simulink model "ALL_IN_ONE"  (R2024b)
settings: Solver=VariableStepAuto  StartTime=0.0  StopTime=0.6  RelTol=1e-3
undefined symbols (not defined in the file or in its folder): sigbuilder_block
libraries: spsSeriesRLCBranchLib x16, spsCurrentMeasurementLib x4, spsDiodeLib x4, spsPWMGeneratorDCDCLib x4, spsMosfetLib x4, spsPVArrayLib x4, spsVoltageMeasurementLib x4, fuzblock x1, deeplib x1, slpidlib x1, spspowerguiLib x1
settings Model: Creator=RASITH  LastModifiedBy=RASITH

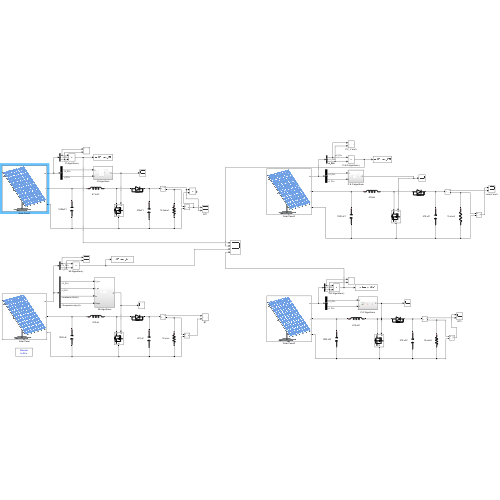
[thumbnail: Simulink's stored preview of the top-level diagram]
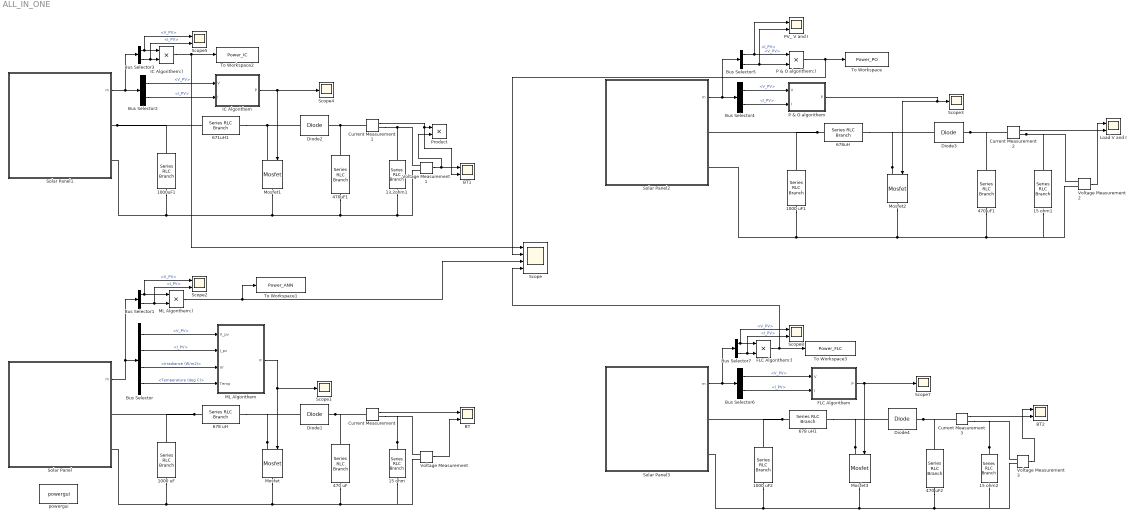
== system ALL_IN_ONE ==
  1000 uF : spsSeriesRLCBranchLib/Series RLC Branch  LConnTagsString=__new0  RConnTagsString=__new0  BranchType=C  Resistance=1  Inductance=1e-3  SetiL0=off  InitialCurrent=0  Capacitance=1e-3  Setx0=off  InitialVoltage=0  Measurements=None
  1000 uF1 : spsSeriesRLCBranchLib/Series RLC Branch  LConnTagsString=__new0  RConnTagsString=__new0  BranchType=C  Resistance=1  Inductance=1e-3  SetiL0=off  InitialCurrent=0  Capacitance=1e-3  Setx0=off  InitialVoltage=0  Measurements=None
  1000 uF2 : spsSeriesRLCBranchLib/Series RLC Branch  LConnTagsString=__new0  RConnTagsString=__new0  BranchType=C  Resistance=1  Inductance=1e-3  SetiL0=off  InitialCurrent=0  Capacitance=1e-3  Setx0=off  InitialVoltage=0  Measurements=None
  1000uF1 : spsSeriesRLCBranchLib/Series RLC Branch  LConnTagsString=__new0  RConnTagsString=__new0  BranchType=C  Resistance=1  Inductance=1e-3  SetiL0=off  InitialCurrent=0  Capacitance=1e-3  Setx0=off  InitialVoltage=0  Measurements=None
  13.2ohm1 : spsSeriesRLCBranchLib/Series RLC Branch  LConnTagsString=__new0  RConnTagsString=__new0  BranchType=R  Resistance=30  Inductance=1e-3  SetiL0=off  InitialCurrent=0  Capacitance=1e-6  Setx0=off  InitialVoltage=0  Measurements=None
  15 ohm : spsSeriesRLCBranchLib/Series RLC Branch  LConnTagsString=__new0  RConnTagsString=__new0  BranchType=R  Resistance=30  Inductance=1e-3  SetiL0=off  InitialCurrent=0  Capacitance=1e-6  Setx0=off  InitialVoltage=0  Measurements=Branch voltage and current
  15 ohm1 : spsSeriesRLCBranchLib/Series RLC Branch  LConnTagsString=__new0  RConnTagsString=__new0  BranchType=R  Resistance=30  Inductance=1e-3  SetiL0=off  InitialCurrent=0  Capacitance=1e-6  Setx0=off  InitialVoltage=0  Measurements=None
  15 ohm2 : spsSeriesRLCBranchLib/Series RLC Branch  LConnTagsString=__new0  RConnTagsString=__new0  BranchType=R  Resistance=17  Inductance=1e-3  SetiL0=off  InitialCurrent=0  Capacitance=1e-6  Setx0=off  InitialVoltage=0  Measurements=None
  470 uF : spsSeriesRLCBranchLib/Series RLC Branch  LConnTagsString=__new0  RConnTagsString=__new0  BranchType=C  Resistance=1  Inductance=1e-3  SetiL0=off  InitialCurrent=0  Capacitance=470e-6  Setx0=off  InitialVoltage=0  Measurements=None
  470 uF1 : spsSeriesRLCBranchLib/Series RLC Branch  LConnTagsString=__new0  RConnTagsString=__new0  BranchType=C  Resistance=1  Inductance=1e-3  SetiL0=off  InitialCurrent=0  Capacitance=470e-6  Setx0=off  InitialVoltage=0  Measurements=None
  470 uF2 : spsSeriesRLCBranchLib/Series RLC Branch  LConnTagsString=__new0  RConnTagsString=__new0  BranchType=C  Resistance=1  Inductance=1e-3  SetiL0=off  InitialCurrent=0  Capacitance=470e-6  Setx0=off  InitialVoltage=40  Measurements=None
  470uF1 : spsSeriesRLCBranchLib/Series RLC Branch  LConnTagsString=__new0  RConnTagsString=__new0  BranchType=C  Resistance=1  Inductance=1e-3  SetiL0=off  InitialCurrent=0  Capacitance=470e-6  Setx0=off  InitialVoltage=0  Measurements=None
  671uH1 : spsSeriesRLCBranchLib/Series RLC Branch  LConnTagsString=__new0  RConnTagsString=__new0  BranchType=L  Resistance=1  Inductance=678e-6  SetiL0=off  InitialCurrent=0  Capacitance=1e-6  Setx0=off  InitialVoltage=0  Measurements=None
  678 uH : spsSeriesRLCBranchLib/Series RLC Branch  LConnTagsString=__new0  RConnTagsString=__new0  BranchType=L  Resistance=1  Inductance=678e-6  SetiL0=off  InitialCurrent=0  Capacitance=1e-6  Setx0=off  InitialVoltage=0  Measurements=None
  678 uH1 : spsSeriesRLCBranchLib/Series RLC Branch  LConnTagsString=__new0  RConnTagsString=__new0  BranchType=L  Resistance=1  Inductance=678e-6  SetiL0=off  InitialCurrent=0  Capacitance=1e-6  Setx0=off  InitialVoltage=0  Measurements=None
  678uH : spsSeriesRLCBranchLib/Series RLC Branch  LConnTagsString=__new0  RConnTagsString=__new0  BranchType=L  Resistance=1  Inductance=678e-6  SetiL0=off  InitialCurrent=0  Capacitance=1e-6  Setx0=off  InitialVoltage=0  Measurements=None
  BT : Scope  NumInputPorts=2
  BT1 : Scope  NumInputPorts=2
  BT2 : Scope  NumInputPorts=2
  Bus Selector : BusSelector  OutputSignals=V_PV,I_PV,Irradiance (W/m2),Temperature (deg C)
  Bus Selector{1..7} (7 alike) : BusSelector  OutputSignals=V_PV,I_PV
  Current Measurement{,1..3} (4 alike) : spsCurrentMeasurementLib/Current Measurement  PhasorSimulation=off  OutputType=Complex  PSBequivalent=0
  Diode{1..4} (4 alike) : spsDiodeLib/Diode  Ron=0.001  Lon=0  Vf=0.8  IC=0  UseSnubber=0  Rs=500  Cs=250e-9  Measurements=off
  FLC Algorithem : Subsystem
  FLC Algorithem:) : Product
  IC Algorithem : Subsystem
  IC Algorithem:) : Product
  Load V and I : Scope  NumInputPorts=2
  ML Algorithem : Subsystem
  ML Algorithem:) : Product
  Mosfet : spsMosfetLib/Mosfet  Ron=4.2e-3  Lon=0  Rd=0.01  Vfd=0  IC=0  Rs=1e5  Cs=1e-9  Measurements=off
  Mosfet1 : spsMosfetLib/Mosfet  Ron=4.2e-3  Lon=0  Rd=0.01  Vfd=0  IC=0  Rs=1e5  Cs=1e-9  Measurements=off
  Mosfet2 : spsMosfetLib/Mosfet  Ron=4.2e-3  Lon=0  Rd=0.01  Vfd=1  IC=0  Rs=1e5  Cs=1e-9  Measurements=off
  Mosfet3 : spsMosfetLib/Mosfet  Ron=4.2e-3  Lon=0  Rd=0.01  Vfd=0  IC=0  Rs=1e5  Cs=1e-9  Measurements=off
  P & O algorithem : Subsystem
  P & O algorithem:) : Product
  PV_ V and I : Scope  NumInputPorts=2
  Product : Product
  Scope : Scope  NumInputPorts=4
  Scope{1,3..4,7} (4 alike) : Scope
  Scope2 : Scope  NumInputPorts=2
  Scope5 : Scope  NumInputPorts=2
  Scope8 : Scope  NumInputPorts=2
  Solar Panel : Subsystem
      mask Display: image('C:\Users\RASITH\MATLAB Drive\Final Year Project [MPPT Boost Converter(PV)]\Solar Panel.png');
  Solar Panel1 : Subsystem
      mask Display: image('C:\Users\RASITH\MATLAB Drive\Final Year Project [MPPT Boost Converter(PV)]\Solar Panel.png');
  Solar Panel2 : Subsystem
      mask Display: image('C:\Users\RASITH\MATLAB Drive\Final Year Project [MPPT Boost Converter(PV)]\Solar Panel.png');
  Solar Panel3 : Subsystem
      mask Display: image('C:\Users\RASITH\MATLAB Drive\Final Year Project [MPPT Boost Converter(PV)]\Solar Panel.png');
  To Workspace : ToWorkspace  VariableName=Power_PO  SaveFormat=Timeseries  SampleTime=-1
  To Workspace1 : ToWorkspace  VariableName=Power_ANN  SaveFormat=Timeseries  SampleTime=-1
  To Workspace2 : ToWorkspace  VariableName=Power_IC  SaveFormat=Timeseries  SampleTime=-1
  To Workspace3 : ToWorkspace  VariableName=Power_FLC  SaveFormat=Timeseries  SampleTime=-1
  Voltage Measurement{,1..3} (4 alike) : spsVoltageMeasurementLib/Voltage Measurement  PhasorSimulation=off  OutputType=Complex  PSBequivalent=0
  powergui : spspowerguiLib/powergui  Priority=1  SimulationMode=Discrete  SampleTime=1e-6  frequency=100000  Iterations=50  frequencyindice=0  Pbase=100e6  ErrMax=1e-4  UnitsV=kV  UnitsW=MW  buscounter=0  FunctionMessages=off  echomessages=off  EnableUseOfTLC=off  CurrentSourceSwitches=off  DisableSnubberDevices=off  DisableRonSwitches=off  DisableVfSwitches=off  DisplayEquations=off  AutomaticDiscreteSolvers=off  SolverType=Tustin/Backward Euler (TBE)  Interpol=off  ExternalGateDelay=off  methode=off  Ts=100  x0status=blocks  SPID=on  SwTol=0  HookPort=off  NonlinearTolerance=1e-4  nMaxIteration=100  ContinueOnMaxIteration=off  RestoreLinks=warning  ResistiveCurrentMeasurement=off  Frange=[0:2:500]  Ylog=off  Xlog=on  ShowGrid=off  save=off  variable=ZData  structure=0  ZoomFFT=off  StartTime=0.0  cycles=1  DisplayStyle=1  fundamental=60  FreqAxis=off  MaxFrequency=1000  frequencyindicesteady=1  RmsSteady=1  display=off
  wires:
  Bus Selector3/1 -> Scope5/1, IC Algorithem:)/1  "<V_PV>"
  Bus Selector/3 -> ML Algorithem/3(Irr)  "<Irradiance (W/m2)>"
  Current Measurement/1 -> BT/1
  Bus Selector3/2 -> Scope5/2, IC Algorithem:)/2  "<I_PV>"
  ML Algorithem:)/1 -> To Workspace1/1, Scope/3
  Current Measurement1/1 -> BT1/2, Product/1
  Voltage Measurement1/1 -> Product/2, BT1/1
  Bus Selector/1 -> ML Algorithem/1(V_pv)  "<V_PV>"
  Bus Selector2/2 -> IC Algorithem/2(I)  "<I_PV>"
  Solar Panel1/1(m) -> Bus Selector3/1, Bus Selector2/1
  IC Algorithem/1(P) -> Scope4/1, Mosfet1/1
  Voltage Measurement/1 -> BT/2
  Bus Selector/4 -> ML Algorithem/4(Temp)  "<Temperature (deg C)>"
  Bus Selector1/2 -> Scope2/2, ML Algorithem:)/2  "<I_PV>"
  Bus Selector1/1 -> Scope2/1, ML Algorithem:)/1  "<V_PV>"
  ML Algorithem/1(P) -> Mosfet/1, Scope1/1
  Solar Panel/1(m) -> Bus Selector1/1, Bus Selector/1
  Bus Selector/2 -> ML Algorithem/2(I_pv)  "<I_PV>"
  Bus Selector2/1 -> IC Algorithem/1(V)  "<V_PV>"
  IC Algorithem:)/1 -> To Workspace2/1, Scope/1
  Bus Selector4/1 -> P & O algorithem/1(V)  "<V_PV>"
  Current Measurement2/1 -> Load V and I/2
  Bus Selector4/2 -> P & O algorithem/2(I)  "<I_PV>"
  Bus Selector5/1 -> PV_ V and I/1, P & O algorithem:)/1  "<V_PV>"
  Bus Selector5/2 -> P & O algorithem:)/2, PV_ V and I/2  "<I_PV>"
  P & O algorithem/1(P) -> Scope3/1, Mosfet2/1
  Solar Panel2/1(m) -> Bus Selector5/1, Bus Selector4/1
  Voltage Measurement2/1 -> Load V and I/1
  Solar Panel3/1(m) -> Bus Selector7/1, Bus Selector6/1
  Bus Selector6/1 -> FLC Algorithem/1(V)  "<V_PV>"
  FLC Algorithem/1(P) -> Scope7/1, Mosfet3/1
  Voltage Measurement3/1 -> BT2/1
  Current Measurement3/1 -> BT2/2
  Bus Selector7/1 -> Scope8/1, FLC Algorithem:)/1  "<V_PV>"
  Bus Selector6/2 -> FLC Algorithem/2(I)  "<I_PV>"
  Bus Selector7/2 -> Scope8/2, FLC Algorithem:)/2  "<I_PV>"
  FLC Algorithem:)/1 -> To Workspace3/1, Scope/4
  P & O algorithem:)/1 -> To Workspace/1, Scope/2
  connections:
  678 uH/LConn1 -- 1000 uF/LConn1 -- Solar Panel/RConn1
  Mosfet/RConn1 -- 15 ohm/RConn1 -- Voltage Measurement/LConn2 -- 470 uF/RConn1 -- 1000 uF/RConn1 -- Solar Panel/RConn2
  Mosfet/LConn1 -- 678 uH/RConn1 -- Diode1/LConn1
  Solar Panel1/RConn1 -- 671uH1/LConn1 -- 1000uF1/LConn1
  Current Measurement1/RConn1 -- 13.2ohm1/LConn1 -- Voltage Measurement1/LConn1
  Diode2/LConn1 -- Mosfet1/LConn1 -- 671uH1/RConn1
  Current Measurement1/LConn1 -- Diode2/RConn1 -- 470uF1/LConn1
  Voltage Measurement1/LConn2 -- 13.2ohm1/RConn1 -- 470uF1/RConn1 -- 1000uF1/RConn1 -- Solar Panel1/RConn2 -- Mosfet1/RConn1
  Diode1/RConn1 -- 470 uF/LConn1 -- Current Measurement/LConn1
  15 ohm/LConn1 -- Voltage Measurement/LConn1 -- Current Measurement/RConn1
  678uH/LConn1 -- 1000 uF1/LConn1 -- Solar Panel2/RConn1
  Mosfet2/RConn1 -- 1000 uF1/RConn1 -- Solar Panel2/RConn2 -- 15 ohm1/RConn1 -- Voltage Measurement2/LConn2 -- 470 uF1/RConn1
  Mosfet2/LConn1 -- 678uH/RConn1 -- Diode3/LConn1
  Diode3/RConn1 -- Current Measurement2/LConn1 -- 470 uF1/LConn1
  Current Measurement2/RConn1 -- Voltage Measurement2/LConn1 -- 15 ohm1/LConn1
  15 ohm2/LConn1 -- Voltage Measurement3/LConn1 -- Current Measurement3/RConn1
  Mosfet3/RConn1 -- Voltage Measurement3/LConn2 -- 15 ohm2/RConn1 -- 470 uF2/RConn1 -- 1000 uF2/RConn1 -- Solar Panel3/RConn2
  Mosfet3/LConn1 -- 678 uH1/RConn1 -- Diode4/LConn1
  Diode4/RConn1 -- 470 uF2/LConn1 -- Current Measurement3/LConn1
  678 uH1/LConn1 -- 1000 uF2/LConn1 -- Solar Panel3/RConn1

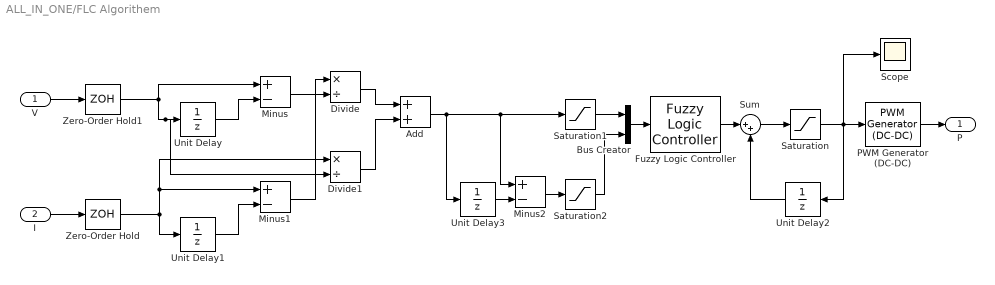
== system ALL_IN_ONE/FLC Algorithem ==
  V : Inport
  I : Inport  Port=2
  Add : Sum
  Bus Creator : BusCreator  Inputs=2
  Divide : Product  Inputs=*/
  Divide1 : Product  Inputs=*/
  Fuzzy Logic Controller : fuzblock/Fuzzy Logic  Controller  FIS=mamdani  OutputSampleNumber=49  DataType=double  FuzzifiedInputs=off  RuleFiringStrengths=off  RuleOutputs=off  AggregatedOutputs=off  SimulateUsing=Interpreted execution  OutOfRangeInputValueMessage=warning  NoRuleFiredMessage=warning  EmptyOutputFuzzySetMessage=warning
  Minus : Sum  Inputs=+-
  Minus1 : Sum  Inputs=+-
  Minus2 : Sum  Inputs=+-
  PWM Generator (DC-DC) : spsPWMGeneratorDCDCLib/PWM Generator (DC-DC)  Fsw=10000  Ts=1e-6
  Saturation : Saturate  UpperLimit=0.9  LowerLimit=0.1
  Saturation1 : Saturate  UpperLimit=1.5  LowerLimit=-1.5
  Saturation2 : Saturate  UpperLimit=0.02  LowerLimit=-0.02
  Scope : Scope
  Sum : Sum  Inputs=|++
  Unit Delay{,1..3} (4 alike) : UnitDelay  SampleTime=-1  HasFrameUpgradeWarning=on
  Zero-Order Hold : ZeroOrderHold  SampleTime=1e-3
  Zero-Order Hold1 : ZeroOrderHold  SampleTime=1e-3
  P : Outport
  wires:
  I/1 -> Zero-Order Hold/1
  V/1 -> Zero-Order Hold1/1
  Bus Creator/1 -> Fuzzy Logic Controller/1
  Fuzzy Logic Controller/1 -> Sum/1
  Sum/1 -> Saturation/1
  Saturation/1 -> Scope/1, PWM Generator (DC-DC)/1, Unit Delay2/1
  Unit Delay2/1 -> Sum/2
  Unit Delay/1 -> Minus/2
  Minus/1 -> Divide/2
  Unit Delay1/1 -> Minus1/2
  Minus1/1 -> Divide/1
  Divide1/1 -> Add/2
  Divide/1 -> Add/1
  PWM Generator (DC-DC)/1 -> P/1
  Add/1 -> Saturation1/1, Minus2/1, Unit Delay3/1
  Saturation1/1 -> Bus Creator/1
  Unit Delay3/1 -> Minus2/2
  Minus2/1 -> Saturation2/1
  Saturation2/1 -> Bus Creator/2
  Zero-Order Hold1/1 -> Divide1/2, Unit Delay/1, Minus/1
  Zero-Order Hold/1 -> Minus1/1, Divide1/1, Unit Delay1/1

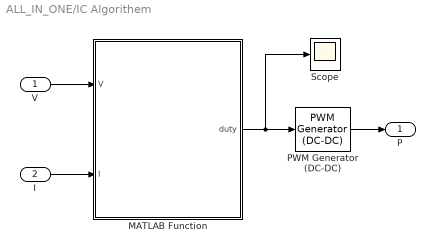
== system ALL_IN_ONE/IC Algorithem ==
  V : Inport
  I : Inport  Port=2
  MATLAB Function : MATLAB Function  TreatAsAtomicUnit=on
  PWM Generator (DC-DC) : spsPWMGeneratorDCDCLib/PWM Generator (DC-DC)  Fsw=10000  Ts=1e-6
  Scope : Scope
  P : Outport
  wires:
  I/1 -> MATLAB Function/2(I)
  V/1 -> MATLAB Function/1(V)
  PWM Generator (DC-DC)/1 -> P/1
  MATLAB Function/1(duty) -> Scope/1, PWM Generator (DC-DC)/1

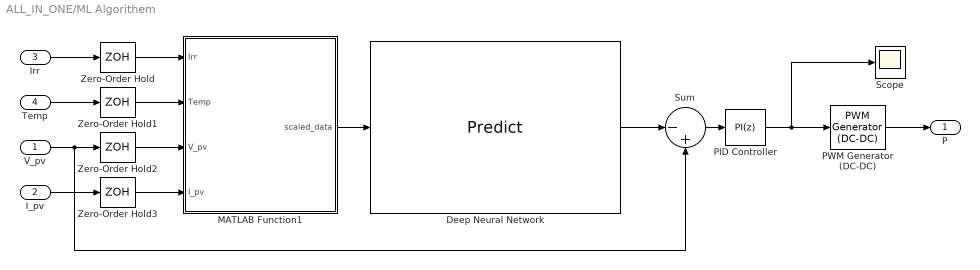
== system ALL_IN_ONE/ML Algorithem ==
  V_pv : Inport
  I_pv : Inport  Port=2
  Irr : Inport  Port=3
  Temp : Inport  Port=4
  Deep Neural Network : deeplib/Predict  Network=Network from MAT-file  NetworkFunction=squeezenet  NetworkFilePath=C:\Users\RASITH\OneDrive - University of Hertfordshire\MPPT\ML\mppt_simulink_model.mat  MiniBatchSize=128  InputDataFormats={'mppt_inputs', 'BC';}  Predictions=on  Activations={}  ForceInterpretedSim=off  EnableDLNetwork=on  LastKnownNetworkFilePath='C:\Users\RASITH\OneDrive - University of Hertfordshire\MPPT\ML\mppt_simulink_model.mat'  LastKnownNetworkTimeStamp=740139.509027777821756899356842041015625
  MATLAB Function1 : MATLAB Function  TreatAsAtomicUnit=on
  PID Controller : slpidlib/PID Controller  Controller=PI  Form=Parallel  TimeDomain=Discrete-time  UseExternalTs=off  SampleTime=-1  IntegratorMethod=Forward Euler  FilterMethod=Forward Euler  ControllerParametersSource=internal  P=0.5  I=6  UseKiTs=off  D=0  UseExternalDerivativeSource=off  N=100  UseFilter=on  TunerSelectOption=Transfer Function Based (PID Tuner App)  InitialConditionSource=internal  InitialConditionForIntegrator=0.5  InitialConditionForFilter=0  DifferentiatorICPrevScaledInput=0  ExternalReset=none  TrackingMode=off  Kt=1  LimitOutput=on  SatLimitsSource=internal  UpperSaturationLimit=0.9  LowerSaturationLimit=0.1  LinearizeAsGain=on  AntiWindupMode=clamping  Kb=1  LimitIntegrator=off  UpperIntegratorSaturationLimit=inf  LowerIntegratorSaturationLimit=-inf  POutMin=[]  POutMax=[]  IOutMin=[]  IOutMax=[]  DOutMin=[]  DOutMax=[]  NOutMin=[]  NOutMax=[]  SumOutMin=[]  SumOutMax=[]  SaturationOutMin=[]  SaturationOutMax=[]  PParamMin=[]  PParamMax=[]  IParamMin=[]  IParamMax=[]  DParamMin=[]  DParamMax=[]  NParamMin=[]  NParamMax=[]  KbParamMin=[]  KbParamMax=[]  KtParamMin=[]  KtParamMax=[]  KbOutMin=[]  KbOutMax=[]  KtOutMin=[]  KtOutMax=[]  IntegratorOutMin=[]  IntegratorOutMax=[]  FilterOutMin=[]  FilterOutMax=[]  SumI1OutMin=[]  SumI1OutMax=[]  SumI2OutMin=[]  SumI2OutMax=[]  SumI3OutMin=[]  SumI3OutMax=[]  SumI4OutMin=[]  SumI4OutMax=[]  SumDOutMin=[]  SumDOutMax=[]  DifferentiatorOutMin=[]  DifferentiatorOutMax=[]  FilterDiffOutCoefMin=[]  FilterDiffOutCoefMax=[]  ReciprocalOutMin=[]  ReciprocalOutMax=[]  SumDenOutMin=[]  SumDenOutMax=[]  SumNumOutMin=[]  SumNumOutMax=[]  DivideOutMin=[]  DivideOutMax=[]  UdiffTsProdOutMin=[]  UdiffTsProdOutMax=[]  NTsProdOutMin=[]  NTsProdOutMax=[]  UintegralTsProdOutMin=[]  UintegralTsProdOutMax=[]  UngainTsProdOutMin=[]  UngainTsProdOutMax=[]  ClampingZeroOutDataTypeStr=Inherit: Inherit via back propagation  ClampingZeroOutMin=[]  ClampingZeroOutMax=[]  FilterDenConstantOutDataTypeStr=Inherit: Inherit via back propagation  FilterDenConstantOutMin=[]  FilterDenConstantOutMax=[]  PCopyOutDataTypeStr=Inherit: Inherit via back propagation  PCopyOutMin=[]  PCopyOutMax=[]  NCopyOutDataTypeStr=Inherit: Inherit via back propagation  NCopyOutMin=[]  NCopyOutMax=[]  IntegratorContinuousStateAttributes=''  IntegratorStateMustResolveToSignalObject=off  IntegratorRTWStateStorageClass=Auto  FilterContinuousStateAttributes=''  FilterStateMustResolveToSignalObject=off  FilterRTWStateStorageClass=Auto  ParallelPVariant=InternalParameters  IdealPVariant=Disabled  IVariant=InternalParameters  DVariant=Disabled  IntegratorVariant=Discrete  SatVariant=Enabled  AWVariant=DiscClampingParallel  PCopyVariant=Disabled  TRVariant=Disabled  FdbkBlocksVariant=Forward  IdealPFdbkVariant=Disabled  SatFdbkVariant=Disabled  DerivativeFilterVariant=Disabled  NVariant=Disabled  NCopyVariant=Disabled_SignalSpec  FilterICVariant=Disabled  IntegratorICVariant=InternalICs  ExternalResetVariant=Disabled  TRSumVariant=Passthrough  SumFdbkVariant=Disabled  SumVariant=Sum_PI  TsampFilterVariant=InternalTs  TsampNgainVariant=Passthrough  TsampIntegralVariant=Disabled_SignalSpec  ExternalSaturationOutDataTypeStr=Inherit: Same as second input  DerivativeSourceVariant=Disabled  PreIntVariant=InternalPreInt
  PWM Generator (DC-DC) : spsPWMGeneratorDCDCLib/PWM Generator (DC-DC)  Fsw=10000  Ts=1e-6
  Scope : Scope
  Sum : Sum  Inputs=|-+
  Zero-Order Hold{,1..3} (4 alike) : ZeroOrderHold  SampleTime=1e-3
  P : Outport
  wires:
  PWM Generator (DC-DC)/1 -> P/1
  MATLAB Function1/1(scaled_data) -> Deep Neural Network/1
  Irr/1 -> Zero-Order Hold/1
  Zero-Order Hold/1 -> MATLAB Function1/1(Irr)
  Temp/1 -> Zero-Order Hold1/1
  I_pv/1 -> Zero-Order Hold3/1
  V_pv/1 -> Sum/2, Zero-Order Hold2/1
  Zero-Order Hold1/1 -> MATLAB Function1/2(Temp)
  Zero-Order Hold2/1 -> MATLAB Function1/3(V_pv)
  Zero-Order Hold3/1 -> MATLAB Function1/4(I_pv)
  PID Controller/1 -> PWM Generator (DC-DC)/1, Scope/1
  Sum/1 -> PID Controller/1
  Deep Neural Network/1 -> Sum/1

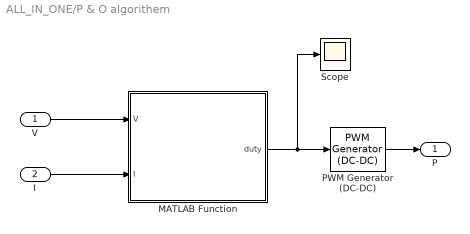
== system ALL_IN_ONE/P & O algorithem ==
  V : Inport
  I : Inport  Port=2
  MATLAB Function : MATLAB Function  TreatAsAtomicUnit=on
  PWM Generator (DC-DC) : spsPWMGeneratorDCDCLib/PWM Generator (DC-DC)  Fsw=10000  Ts=1e-6
  Scope : Scope
  P : Outport
  wires:
  I/1 -> MATLAB Function/2(I)
  V/1 -> MATLAB Function/1(V)
  PWM Generator (DC-DC)/1 -> P/1
  MATLAB Function/1(duty) -> PWM Generator (DC-DC)/1, Scope/1

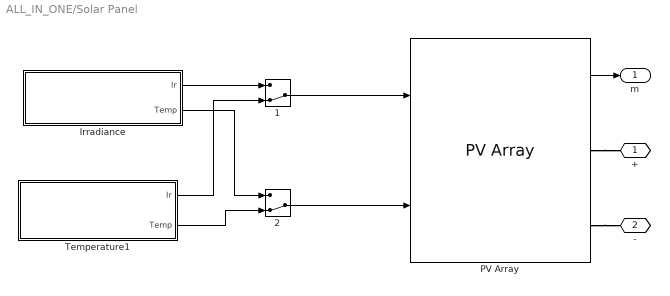
== system ALL_IN_ONE/Solar Panel ==
  "      1" : ManualSwitch  CurrentSetting=0
  "      2" : ManualSwitch  CurrentSetting=0
  "Irradiance " : Subsystem  Tag=STV Subsys  LoadFcn=sigbuilder_block('load');  StartFcn=sigbuilder_block('start');  StopFcn=sigbuilder_block('stop');  ClipboardFcn=sigbuilder_block('clipboard');  mask(Sigbuilder block){tuvar=[0:10]}
      mask help: Sigbuilder GUI
      mask init:
      | if ~strcmp(get_param(bdroot(gcbh),'SimulationStatus'),'stopped') tuvar = sigbuilder_block('maskInit'); end
      settings: CopyFcn=sigbuilder_block('copy');  DeleteFcn=sigbuilder_block('delete');  ModelCloseFcn=sigbuilder_block('modelClose');  PreSaveFcn=sigbuilder_block('preSave');  PauseFcn=sigbuilder_block('pause')  ContinueFcn=sigbuilder_block('continue')  NameChangeFcn=sigbuilder_block('namechange');  OpenFcn=sigbuilder_block('open',[118.2 99 596.4 429.6 ]);  CloseFcn=sigbuilder_block('close');
      mask Display: plot(0, 0, 100, 100,[2, 2, 32, 32, 2], [68, 8, 8, 68, 68],[32, 2], [38, 38], [32, 19, 2],[53, 60, 44], [32, 17, 17, 2],[16, 16, 31, 31]);txt = getActiveGroup(gcbh);text(2, 100, txt,'verticalAlignment', 'top');
  PV Array : spsPVArrayLib/PV Array  Npar=1  Nser=1  PlotType=array @ 1000 W/m2 & specified temperatures  S_vec="[ 1000  500  100 ]"  Temp_C_vec="[ 25  ]"  ModuleName=User-defined  PlotWhenSelected=off  Pm=50.04  Ncell=36  Voc=23.4  Isc=2.92  Vm=18  Im=2.78  beta_Voc_pc=-0.36099  alpha_Isc_pc=0.102  beta_Voc=-0.084472  alpha_Isc=0.0029784  IL=2.9466  I0=1.0988e-10  nI=1.0538  Rsh=1848.6949  Rs=0.95616  RobustModel=off  RobustCellTemperature=313.3991  BAL=on  Tc=1e-6  Tfilter=5e-5
  Temperature1 : Subsystem  Tag=STV Subsys  LoadFcn=sigbuilder_block('load');  StartFcn=sigbuilder_block('start');  StopFcn=sigbuilder_block('stop');  ClipboardFcn=sigbuilder_block('clipboard');  mask(Sigbuilder block){tuvar=[0:10]}
      mask help: Sigbuilder GUI
      mask init:
      | if ~strcmp(get_param(bdroot(gcbh),'SimulationStatus'),'stopped') tuvar = sigbuilder_block('maskInit'); end
      settings: CopyFcn=sigbuilder_block('copy');  DeleteFcn=sigbuilder_block('delete');  ModelCloseFcn=sigbuilder_block('modelClose');  PreSaveFcn=sigbuilder_block('preSave');  PauseFcn=sigbuilder_block('pause')  ContinueFcn=sigbuilder_block('continue')  NameChangeFcn=sigbuilder_block('namechange');  OpenFcn=sigbuilder_block('open',[5.4 36 1141.2 516.6 ]);  CloseFcn=sigbuilder_block('close');
      mask Display: plot(0, 0, 100, 100,[2, 2, 32, 32, 2], [68, 8, 8, 68, 68],[32, 2], [38, 38], [32, 19, 2],[53, 60, 44], [32, 17, 17, 2],[16, 16, 31, 31]);txt = getActiveGroup(gcbh);text(2, 100, txt,'verticalAlignment', 'top');
  + : PMIOPort  Side=Right
  - : PMIOPort  Port=2  Side=Right
  m : Outport
  wires:
  "Irradiance "/1(Ir) -> "      1"/1
  "      2"/1 -> PV Array/2
  "      1"/1 -> PV Array/1
  Temperature1/2(Temp) -> "      2"/2
  Temperature1/1(Ir) -> "      1"/2
  "Irradiance "/2(Temp) -> "      2"/1
  PV Array/1 -> m/1
  connections:
  PV Array/RConn1 -- +/RConn1
  PV Array/RConn2 -- -/RConn1

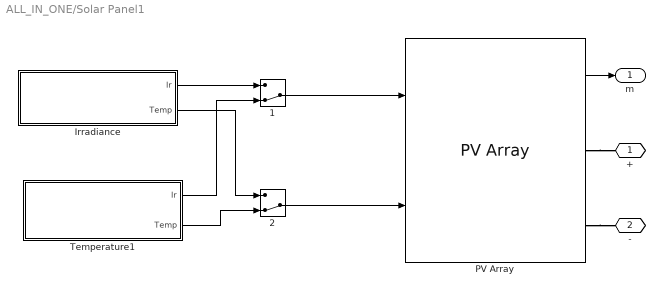
== system ALL_IN_ONE/Solar Panel1 ==
  "      1" : ManualSwitch  CurrentSetting=0
  "      2" : ManualSwitch  CurrentSetting=0
  "Irradiance " : Subsystem  Tag=STV Subsys  LoadFcn=sigbuilder_block('load');  StartFcn=sigbuilder_block('start');  StopFcn=sigbuilder_block('stop');  ClipboardFcn=sigbuilder_block('clipboard');  mask(Sigbuilder block){tuvar=[0:10]}
      mask help: Sigbuilder GUI
      mask init:
      | if ~strcmp(get_param(bdroot(gcbh),'SimulationStatus'),'stopped') tuvar = sigbuilder_block('maskInit'); end
      settings: CopyFcn=sigbuilder_block('copy');  DeleteFcn=sigbuilder_block('delete');  ModelCloseFcn=sigbuilder_block('modelClose');  PreSaveFcn=sigbuilder_block('preSave');  PauseFcn=sigbuilder_block('pause')  ContinueFcn=sigbuilder_block('continue')  NameChangeFcn=sigbuilder_block('namechange');  OpenFcn=sigbuilder_block('open',[150 94.8 596.4 429.6 ]);  CloseFcn=sigbuilder_block('close');
      mask Display: plot(0, 0, 100, 100,[2, 2, 32, 32, 2], [68, 8, 8, 68, 68],[32, 2], [38, 38], [32, 19, 2],[53, 60, 44], [32, 17, 17, 2],[16, 16, 31, 31]);txt = getActiveGroup(gcbh);text(2, 100, txt,'verticalAlignment', 'top');
  PV Array : spsPVArrayLib/PV Array  Npar=1  Nser=1  PlotType=array @ 1000 W/m2 & specified temperatures  S_vec="[ 1000  500  100 ]"  Temp_C_vec="[ 25  ]"  ModuleName=User-defined  PlotWhenSelected=off  Pm=50.04  Ncell=36  Voc=23.4  Isc=2.92  Vm=18  Im=2.78  beta_Voc_pc=-0.36099  alpha_Isc_pc=0.102  beta_Voc=-0.084472  alpha_Isc=0.0029784  IL=2.9466  I0=1.0988e-10  nI=1.0538  Rsh=1848.6949  Rs=0.95616  RobustModel=off  RobustCellTemperature=313.3991  BAL=on  Tc=1e-6  Tfilter=5e-5
  Temperature1 : Subsystem  Tag=STV Subsys  LoadFcn=sigbuilder_block('load');  StartFcn=sigbuilder_block('start');  StopFcn=sigbuilder_block('stop');  ClipboardFcn=sigbuilder_block('clipboard');  mask(Sigbuilder block){tuvar=[0:10]}
      mask help: Sigbuilder GUI
      mask init:
      | if ~strcmp(get_param(bdroot(gcbh),'SimulationStatus'),'stopped') tuvar = sigbuilder_block('maskInit'); end
      settings: CopyFcn=sigbuilder_block('copy');  DeleteFcn=sigbuilder_block('delete');  ModelCloseFcn=sigbuilder_block('modelClose');  PreSaveFcn=sigbuilder_block('preSave');  PauseFcn=sigbuilder_block('pause')  ContinueFcn=sigbuilder_block('continue')  NameChangeFcn=sigbuilder_block('namechange');  OpenFcn=sigbuilder_block('open',[130.2 54 909.6 516.6 ]);  CloseFcn=sigbuilder_block('close');
      mask Display: plot(0, 0, 100, 100,[2, 2, 32, 32, 2], [68, 8, 8, 68, 68],[32, 2], [38, 38], [32, 19, 2],[53, 60, 44], [32, 17, 17, 2],[16, 16, 31, 31]);txt = getActiveGroup(gcbh);text(2, 100, txt,'verticalAlignment', 'top');
  + : PMIOPort  Side=Right
  - : PMIOPort  Port=2  Side=Right
  m : Outport
  wires:
  "Irradiance "/1(Ir) -> "      1"/1
  "      2"/1 -> PV Array/2
  "      1"/1 -> PV Array/1
  Temperature1/2(Temp) -> "      2"/2
  Temperature1/1(Ir) -> "      1"/2
  "Irradiance "/2(Temp) -> "      2"/1
  PV Array/1 -> m/1
  connections:
  PV Array/RConn1 -- +/RConn1
  PV Array/RConn2 -- -/RConn1

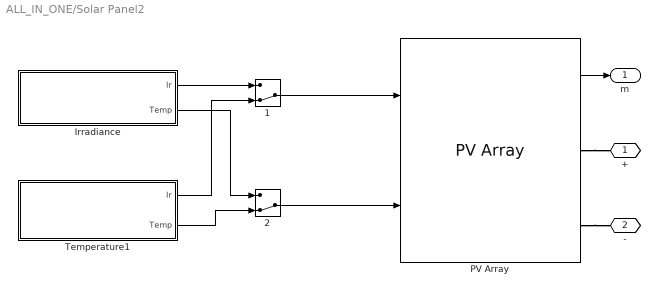
== system ALL_IN_ONE/Solar Panel2 ==
  "      1" : ManualSwitch  CurrentSetting=0
  "      2" : ManualSwitch  CurrentSetting=0
  "Irradiance " : Subsystem  Tag=STV Subsys  LoadFcn=sigbuilder_block('load');  StartFcn=sigbuilder_block('start');  StopFcn=sigbuilder_block('stop');  ClipboardFcn=sigbuilder_block('clipboard');  mask(Sigbuilder block){tuvar=[0:10]}
      mask help: Sigbuilder GUI
      mask init:
      | if ~strcmp(get_param(bdroot(gcbh),'SimulationStatus'),'stopped') tuvar = sigbuilder_block('maskInit'); end
      settings: CopyFcn=sigbuilder_block('copy');  DeleteFcn=sigbuilder_block('delete');  ModelCloseFcn=sigbuilder_block('modelClose');  PreSaveFcn=sigbuilder_block('preSave');  PauseFcn=sigbuilder_block('pause')  ContinueFcn=sigbuilder_block('continue')  NameChangeFcn=sigbuilder_block('namechange');  OpenFcn=sigbuilder_block('open',[118.2 99 596.4 429.6 ]);  CloseFcn=sigbuilder_block('close');
      mask Display: plot(0, 0, 100, 100,[2, 2, 32, 32, 2], [68, 8, 8, 68, 68],[32, 2], [38, 38], [32, 19, 2],[53, 60, 44], [32, 17, 17, 2],[16, 16, 31, 31]);txt = getActiveGroup(gcbh);text(2, 100, txt,'verticalAlignment', 'top');
  PV Array : spsPVArrayLib/PV Array  Npar=1  Nser=1  PlotType=array @ 1000 W/m2 & specified temperatures  S_vec="[ 1000  500  100 ]"  Temp_C_vec="[ 25  ]"  ModuleName=User-defined  PlotWhenSelected=off  Pm=50.04  Ncell=36  Voc=23.4  Isc=2.92  Vm=18  Im=2.78  beta_Voc_pc=-0.36099  alpha_Isc_pc=0.102  beta_Voc=-0.084472  alpha_Isc=0.0029784  IL=2.9466  I0=1.0988e-10  nI=1.0538  Rsh=1848.6949  Rs=0.95616  RobustModel=off  RobustCellTemperature=313.3991  BAL=on  Tc=1e-6  Tfilter=5e-5
  Temperature1 : Subsystem  Tag=STV Subsys  LoadFcn=sigbuilder_block('load');  StartFcn=sigbuilder_block('start');  StopFcn=sigbuilder_block('stop');  ClipboardFcn=sigbuilder_block('clipboard');  mask(Sigbuilder block){tuvar=[0:10]}
      mask help: Sigbuilder GUI
      mask init:
      | if ~strcmp(get_param(bdroot(gcbh),'SimulationStatus'),'stopped') tuvar = sigbuilder_block('maskInit'); end
      settings: CopyFcn=sigbuilder_block('copy');  DeleteFcn=sigbuilder_block('delete');  ModelCloseFcn=sigbuilder_block('modelClose');  PreSaveFcn=sigbuilder_block('preSave');  PauseFcn=sigbuilder_block('pause')  ContinueFcn=sigbuilder_block('continue')  NameChangeFcn=sigbuilder_block('namechange');  OpenFcn=sigbuilder_block('open',[5.4 36 1141.2 516.6 ]);  CloseFcn=sigbuilder_block('close');
      mask Display: plot(0, 0, 100, 100,[2, 2, 32, 32, 2], [68, 8, 8, 68, 68],[32, 2], [38, 38], [32, 19, 2],[53, 60, 44], [32, 17, 17, 2],[16, 16, 31, 31]);txt = getActiveGroup(gcbh);text(2, 100, txt,'verticalAlignment', 'top');
  + : PMIOPort  Side=Right
  - : PMIOPort  Port=2  Side=Right
  m : Outport
  wires:
  "Irradiance "/1(Ir) -> "      1"/1
  "      2"/1 -> PV Array/2
  "      1"/1 -> PV Array/1
  Temperature1/2(Temp) -> "      2"/2
  Temperature1/1(Ir) -> "      1"/2
  "Irradiance "/2(Temp) -> "      2"/1
  PV Array/1 -> m/1
  connections:
  PV Array/RConn1 -- +/RConn1
  PV Array/RConn2 -- -/RConn1

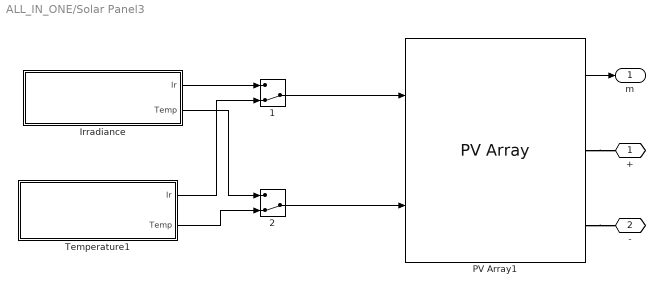
== system ALL_IN_ONE/Solar Panel3 ==
  "      1" : ManualSwitch  CurrentSetting=0
  "      2" : ManualSwitch  CurrentSetting=0
  "Irradiance " : Subsystem  Tag=STV Subsys  LoadFcn=sigbuilder_block('load');  StartFcn=sigbuilder_block('start');  StopFcn=sigbuilder_block('stop');  ClipboardFcn=sigbuilder_block('clipboard');  mask(Sigbuilder block){tuvar=[0:10]}
      mask help: Sigbuilder GUI
      mask init:
      | if ~strcmp(get_param(bdroot(gcbh),'SimulationStatus'),'stopped') tuvar = sigbuilder_block('maskInit'); end
      settings: CopyFcn=sigbuilder_block('copy');  DeleteFcn=sigbuilder_block('delete');  ModelCloseFcn=sigbuilder_block('modelClose');  PreSaveFcn=sigbuilder_block('preSave');  PauseFcn=sigbuilder_block('pause')  ContinueFcn=sigbuilder_block('continue')  NameChangeFcn=sigbuilder_block('namechange');  OpenFcn=sigbuilder_block('open',[118.2 99 596.4 429.6 ]);  CloseFcn=sigbuilder_block('close');
      mask Display: plot(0, 0, 100, 100,[2, 2, 32, 32, 2], [68, 8, 8, 68, 68],[32, 2], [38, 38], [32, 19, 2],[53, 60, 44], [32, 17, 17, 2],[16, 16, 31, 31]);txt = getActiveGroup(gcbh);text(2, 100, txt,'verticalAlignment', 'top');
  PV Array1 : spsPVArrayLib/PV Array  Npar=1  Nser=1  PlotType=array @ 1000 W/m2 & specified temperatures  S_vec="[ 1000  500  100 ]"  Temp_C_vec="[ 25  ]"  ModuleName=User-defined  PlotWhenSelected=off  Pm=50.04  Ncell=36  Voc=23.4  Isc=2.92  Vm=18  Im=2.78  beta_Voc_pc=-0.36099  alpha_Isc_pc=0.102  beta_Voc=-0.084472  alpha_Isc=0.0029784  IL=2.9466  I0=1.0988e-10  nI=1.0538  Rsh=1848.6949  Rs=0.95616  RobustModel=off  RobustCellTemperature=313.3991  BAL=on  Tc=1e-6  Tfilter=5e-5
  Temperature1 : Subsystem  Tag=STV Subsys  LoadFcn=sigbuilder_block('load');  StartFcn=sigbuilder_block('start');  StopFcn=sigbuilder_block('stop');  ClipboardFcn=sigbuilder_block('clipboard');  mask(Sigbuilder block){tuvar=[0:10]}
      mask help: Sigbuilder GUI
      mask init:
      | if ~strcmp(get_param(bdroot(gcbh),'SimulationStatus'),'stopped') tuvar = sigbuilder_block('maskInit'); end
      settings: CopyFcn=sigbuilder_block('copy');  DeleteFcn=sigbuilder_block('delete');  ModelCloseFcn=sigbuilder_block('modelClose');  PreSaveFcn=sigbuilder_block('preSave');  PauseFcn=sigbuilder_block('pause')  ContinueFcn=sigbuilder_block('continue')  NameChangeFcn=sigbuilder_block('namechange');  OpenFcn=sigbuilder_block('open',[5.4 36 1141.2 516.6 ]);  CloseFcn=sigbuilder_block('close');
      mask Display: plot(0, 0, 100, 100,[2, 2, 32, 32, 2], [68, 8, 8, 68, 68],[32, 2], [38, 38], [32, 19, 2],[53, 60, 44], [32, 17, 17, 2],[16, 16, 31, 31]);txt = getActiveGroup(gcbh);text(2, 100, txt,'verticalAlignment', 'top');
  + : PMIOPort  Side=Right
  - : PMIOPort  Port=2  Side=Right
  m : Outport
  wires:
  "Irradiance "/1(Ir) -> "      1"/1
  "      2"/1 -> PV Array1/2
  "      1"/1 -> PV Array1/1
  Temperature1/2(Temp) -> "      2"/2
  Temperature1/1(Ir) -> "      1"/2
  "Irradiance "/2(Temp) -> "      2"/1
  PV Array1/1 -> m/1
  connections:
  PV Array1/RConn1 -- +/RConn1
  PV Array1/RConn2 -- -/RConn1

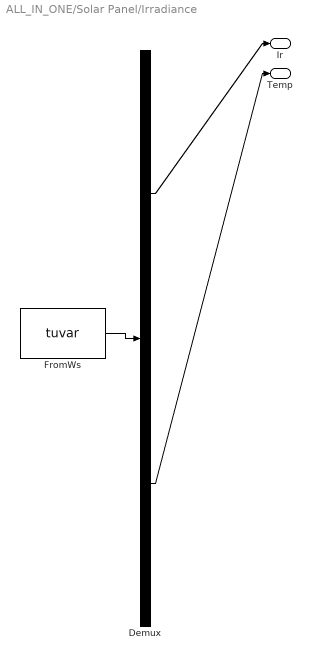
== system ALL_IN_ONE/Solar Panel/Irradiance  ==
  Demux : Demux  Tag=STV Demux  Outputs=2
      settings: DisplayOption=none
  FromWs : FromWorkspace  Tag=STV FromWs  VariableName=tuvar
      SigBuilderData=|
      | common.afterFinalStr = 'Extrapolate'
      | common.sampleTime = '0'
      | dataSet(1).timeRange = [0 2]
      | dataSet(1).name = 'Constant Irradiance'
      | dataSet(2).timeRange = [0 2]
      | dataSet(2).name = 'Step Irradiance'
      | dataSet(3).timeRange = [0 1]
      | dataSet(3).name = 'Ramp-up/down Irradiance'
      | sbobj.Groups(1).Name = 'Constant Irradiance'
      | sbobj.Groups(1).Signals(1).Name = 'Ir'
      | sbobj.Groups(1).Signals(1).XData = [0 2]
      | sbobj.Groups(1).Signals(1).YData = [1000 1000]
      | sbobj.Groups(1).Signals(2).Name = 'Temp'
      | sbobj.Groups(1).Signals(2).XData = [0 1 1 2]
      | sbobj.Groups(1).Signals(2).YData = [0 0 1 1]
      | sbobj.Groups(1).TimeRange = [0 2]
      | sbobj.Groups(2).Name = 'Step Irradiance'
      | sbobj.Groups(2).Signals(1).Name = 'Ir'
      | sbobj.Groups(2).Signals(1).XData = [0 0.252 0.252 2]
      | sbobj.Groups(2).Signals(1).YData = [600 600 1000 1000]
      | sbobj.Groups(2).Signals(2).Name = 'Temp'
      | sbobj.Groups(2).Signals(2).XData = [0 1 1 2]
      | sbobj.Groups(2).Signals(2).YData = [0 0 1 1]
      | sbobj.Groups(2).TimeRange = [0 2]
      | sbobj.Groups(3).Name = 'Ramp-up/down Irradiance'
      | sbobj.Groups(3).Signals(1).Name = 'Ir'
      | sbobj.Groups(3).Signals(1).XData = [0 0.2 0.2 0.4 0.4 0.6 0.6 0.8 0.8 1]
      | sbobj.Groups(3).Signals(1).YData = [1000 1000 100 100 400 400 700 700 1000 1000]
      | sbobj.Groups(3).Signals(2).Name = 'Temp'
      | sbobj.Groups(3).Signals(2).XData = [0 1]
      | sbobj.Groups(3).Signals(2).YData = [25 25]
      | sbobj.Groups(3).TimeRange = [0 1]
  Ir : Outport  Tag=STV Outport
  Temp : Outport  Tag=STV Outport  Port=2
  wires:
  Demux/1 -> Ir/1
  FromWs/1 -> Demux/1
  Demux/2 -> Temp/1

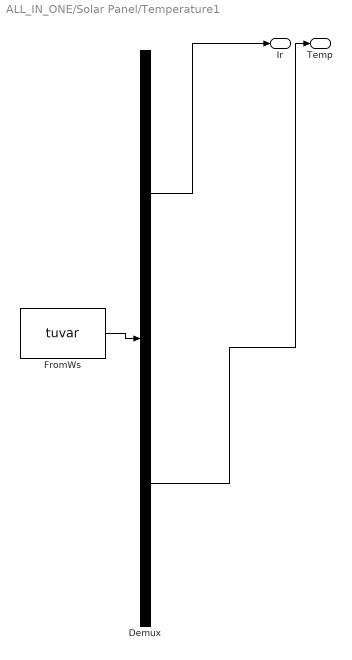
== system ALL_IN_ONE/Solar Panel/Temperature1 ==
  Demux : Demux  Tag=STV Demux  Outputs=2
      settings: DisplayOption=none
  FromWs : FromWorkspace  Tag=STV FromWs  VariableName=tuvar
      SigBuilderData=|
      | common.afterFinalStr = 'Extrapolate'
      | common.sampleTime = '0'
      | dataSet(1).timeRange = [0 1]
      | dataSet(1).name = 'Constant Irradiance'
      | dataSet(2).timeRange = [0 2]
      | dataSet(2).name = 'Ramp-up/down Irradiance'
      | dataSet(3).timeRange = [0 2]
      | dataSet(3).name = 'Step Irradiance'
      | sbobj.Groups(1).Name = 'Constant Irradiance'
      | sbobj.Groups(1).Signals(1).Name = 'Ir'
      | sbobj.Groups(1).Signals(1).XData = [0 1]
      | sbobj.Groups(1).Signals(1).YData = [1000 1000]
      | sbobj.Groups(1).Signals(2).Name = 'Temp'
      | sbobj.Groups(1).Signals(2).XData = [0 0.2 0.2 0.4 0.4 1]
      | sbobj.Groups(1).Signals(2).YData = [25 25 45 45 60 60]
      | sbobj.Groups(1).TimeRange = [0 1]
      | sbobj.Groups(2).Name = 'Ramp-up/down Irradiance'
      | sbobj.Groups(2).Signals(1).Name = 'Ir'
      | sbobj.Groups(2).Signals(1).XData = [0 0.3 0.3 0.4 0.4 0.5 0.5 1 2]
      | sbobj.Groups(2).Signals(1).YData = [1000 1000 800 795 600 600 400 395 395]
      | sbobj.Groups(2).Signals(2).Name = 'Temp'
      | sbobj.Groups(2).Signals(2).XData = [0 0.8 0.8 2]
      | sbobj.Groups(2).Signals(2).YData = [15 15 35 35]
      | sbobj.Groups(2).TimeRange = [0 2]
      | sbobj.Groups(3).Name = 'Step Irradiance'
      | sbobj.Groups(3).Signals(1).Name = 'Ir'
      | sbobj.Groups(3).Signals(1).XData = [0 0.252 0.252 2]
      | sbobj.Groups(3).Signals(1).YData = [600 600 1000 1000]
      | sbobj.Groups(3).Signals(2).Name = 'Temp'
      | sbobj.Groups(3).Signals(2).XData = [0 0.6 0.6 2]
      | sbobj.Groups(3).Signals(2).YData = [15 15 36.5 19.5]
      | sbobj.Groups(3).TimeRange = [0 2]
  Ir : Outport  Tag=STV Outport
  Temp : Outport  Tag=STV Outport  Port=2
  wires:
  FromWs/1 -> Demux/1
  Demux/1 -> Ir/1
  Demux/2 -> Temp/1

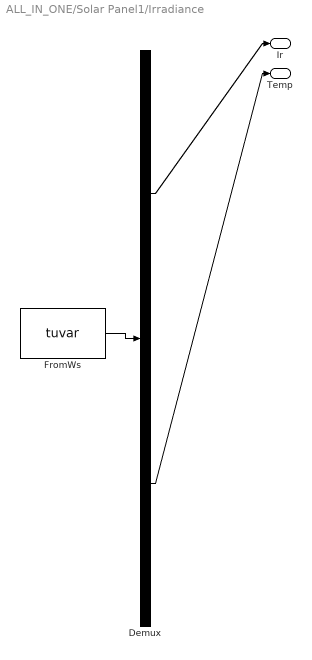
== system ALL_IN_ONE/Solar Panel1/Irradiance  ==
  Demux : Demux  Tag=STV Demux  Outputs=2
      settings: DisplayOption=none
  FromWs : FromWorkspace  Tag=STV FromWs  VariableName=tuvar
      SigBuilderData=|
      | common.afterFinalStr = 'Extrapolate'
      | common.sampleTime = '0'
      | dataSet(1).timeRange = [0 2]
      | dataSet(1).name = 'Constant Irradiance'
      | dataSet(2).timeRange = [0 2]
      | dataSet(2).name = 'Step Irradiance'
      | dataSet(3).timeRange = [0 1]
      | dataSet(3).name = 'Ramp-up/down Irradiance'
      | sbobj.Groups(1).Name = 'Constant Irradiance'
      | sbobj.Groups(1).Signals(1).Name = 'Ir'
      | sbobj.Groups(1).Signals(1).XData = [0 2]
      | sbobj.Groups(1).Signals(1).YData = [1000 1000]
      | sbobj.Groups(1).Signals(2).Name = 'Temp'
      | sbobj.Groups(1).Signals(2).XData = [0 1 1 2]
      | sbobj.Groups(1).Signals(2).YData = [0 0 1 1]
      | sbobj.Groups(1).TimeRange = [0 2]
      | sbobj.Groups(2).Name = 'Step Irradiance'
      | sbobj.Groups(2).Signals(1).Name = 'Ir'
      | sbobj.Groups(2).Signals(1).XData = [0 0.252 0.252 2]
      | sbobj.Groups(2).Signals(1).YData = [600 600 1000 1000]
      | sbobj.Groups(2).Signals(2).Name = 'Temp'
      | sbobj.Groups(2).Signals(2).XData = [0 1 1 2]
      | sbobj.Groups(2).Signals(2).YData = [0 0 1 1]
      | sbobj.Groups(2).TimeRange = [0 2]
      | sbobj.Groups(3).Name = 'Ramp-up/down Irradiance'
      | sbobj.Groups(3).Signals(1).Name = 'Ir'
      | sbobj.Groups(3).Signals(1).XData = [0 0.2 0.2 0.4 0.4 0.6 0.6 0.8 0.8 1]
      | sbobj.Groups(3).Signals(1).YData = [1000 1000 100 100 400 400 700 700 1000 1000]
      | sbobj.Groups(3).Signals(2).Name = 'Temp'
      | sbobj.Groups(3).Signals(2).XData = [0 1]
      | sbobj.Groups(3).Signals(2).YData = [25 25]
      | sbobj.Groups(3).TimeRange = [0 1]
  Ir : Outport  Tag=STV Outport
  Temp : Outport  Tag=STV Outport  Port=2
  wires:
  Demux/1 -> Ir/1
  FromWs/1 -> Demux/1
  Demux/2 -> Temp/1

== system ALL_IN_ONE/Solar Panel1/Temperature1 ==
  Demux : Demux  Tag=STV Demux  Outputs=2
      settings: DisplayOption=none
  FromWs : FromWorkspace  Tag=STV FromWs  VariableName=tuvar
      SigBuilderData=|
      | common.afterFinalStr = 'Extrapolate'
      | common.sampleTime = '0'
      | dataSet(1).timeRange = [0 1]
      | dataSet(1).name = 'Constant Irradiance'
      | dataSet(2).timeRange = [0 2]
      | dataSet(2).name = 'Ramp-up/down Irradiance'
      | dataSet(3).timeRange = [0 2]
      | dataSet(3).name = 'Step Irradiance'
      | sbobj.Groups(1).Name = 'Constant Irradiance'
      | sbobj.Groups(1).Signals(1).Name = 'Ir'
      | sbobj.Groups(1).Signals(1).XData = [0 1]
      | sbobj.Groups(1).Signals(1).YData = [1000 1000]
      | sbobj.Groups(1).Signals(2).Name = 'Temp'
      | sbobj.Groups(1).Signals(2).XData = [0 0.325 0.325 0.675 0.675 1]
      | sbobj.Groups(1).Signals(2).YData = [25 25 45 45 60 60]
      | sbobj.Groups(1).TimeRange = [0 1]
      | sbobj.Groups(2).Name = 'Ramp-up/down Irradiance'
      | sbobj.Groups(2).Signals(1).Name = 'Ir'
      | sbobj.Groups(2).Signals(1).XData = [0 0.3 0.3 0.4 0.4 0.5 0.5 1 2]
      | sbobj.Groups(2).Signals(1).YData = [1000 1000 800 795 600 600 400 395 395]
      | sbobj.Groups(2).Signals(2).Name = 'Temp'
      | sbobj.Groups(2).Signals(2).XData = [0 0.8 0.8 2]
      | sbobj.Groups(2).Signals(2).YData = [15 15 35 35]
      | sbobj.Groups(2).TimeRange = [0 2]
      | sbobj.Groups(3).Name = 'Step Irradiance'
      | sbobj.Groups(3).Signals(1).Name = 'Ir'
      | sbobj.Groups(3).Signals(1).XData = [0 0.252 0.252 2]
      | sbobj.Groups(3).Signals(1).YData = [600 600 1000 1000]
      | sbobj.Groups(3).Signals(2).Name = 'Temp'
      | sbobj.Groups(3).Signals(2).XData = [0 0.6 0.6 2]
      | sbobj.Groups(3).Signals(2).YData = [15 15 36.5 19.5]
      | sbobj.Groups(3).TimeRange = [0 2]
  Ir : Outport  Tag=STV Outport
  Temp : Outport  Tag=STV Outport  Port=2
  wires:
  FromWs/1 -> Demux/1
  Demux/1 -> Ir/1
  Demux/2 -> Temp/1

== system ALL_IN_ONE/Solar Panel2/Irradiance  ==
  Demux : Demux  Tag=STV Demux  Outputs=2
      settings: DisplayOption=none
  FromWs : FromWorkspace  Tag=STV FromWs  VariableName=tuvar
      SigBuilderData=|
      | common.afterFinalStr = 'Extrapolate'
      | common.sampleTime = '0'
      | dataSet(1).timeRange = [0 2]
      | dataSet(1).name = 'Constant Irradiance'
      | dataSet(2).timeRange = [0 2]
      | dataSet(2).name = 'Step Irradiance'
      | dataSet(3).timeRange = [0 1]
      | dataSet(3).name = 'Ramp-up/down Irradiance'
      | sbobj.Groups(1).Name = 'Constant Irradiance'
      | sbobj.Groups(1).Signals(1).Name = 'Ir'
      | sbobj.Groups(1).Signals(1).XData = [0 2]
      | sbobj.Groups(1).Signals(1).YData = [1000 1000]
      | sbobj.Groups(1).Signals(2).Name = 'Temp'
      | sbobj.Groups(1).Signals(2).XData = [0 1 1 2]
      | sbobj.Groups(1).Signals(2).YData = [0 0 1 1]
      | sbobj.Groups(1).TimeRange = [0 2]
      | sbobj.Groups(2).Name = 'Step Irradiance'
      | sbobj.Groups(2).Signals(1).Name = 'Ir'
      | sbobj.Groups(2).Signals(1).XData = [0 0.252 0.252 2]
      | sbobj.Groups(2).Signals(1).YData = [600 600 1000 1000]
      | sbobj.Groups(2).Signals(2).Name = 'Temp'
      | sbobj.Groups(2).Signals(2).XData = [0 1 1 2]
      | sbobj.Groups(2).Signals(2).YData = [0 0 1 1]
      | sbobj.Groups(2).TimeRange = [0 2]
      | sbobj.Groups(3).Name = 'Ramp-up/down Irradiance'
      | sbobj.Groups(3).Signals(1).Name = 'Ir'
      | sbobj.Groups(3).Signals(1).XData = [0 0.2 0.2 0.4 0.4 0.6 0.6 0.8 0.8 1]
      | sbobj.Groups(3).Signals(1).YData = [1000 1000 100 100 400 400 700 700 1000 1000]
      | sbobj.Groups(3).Signals(2).Name = 'Temp'
      | sbobj.Groups(3).Signals(2).XData = [0 1]
      | sbobj.Groups(3).Signals(2).YData = [25 25]
      | sbobj.Groups(3).TimeRange = [0 1]
  Ir : Outport  Tag=STV Outport
  Temp : Outport  Tag=STV Outport  Port=2
  wires:
  Demux/1 -> Ir/1
  FromWs/1 -> Demux/1
  Demux/2 -> Temp/1

== system ALL_IN_ONE/Solar Panel2/Temperature1 ==
  Demux : Demux  Tag=STV Demux  Outputs=2
      settings: DisplayOption=none
  FromWs : FromWorkspace  Tag=STV FromWs  VariableName=tuvar
      SigBuilderData=|
      | common.afterFinalStr = 'Extrapolate'
      | common.sampleTime = '0'
      | dataSet(1).timeRange = [0 1]
      | dataSet(1).name = 'Constant Irradiance'
      | dataSet(2).timeRange = [0 2]
      | dataSet(2).name = 'Ramp-up/down Irradiance'
      | dataSet(3).timeRange = [0 2]
      | dataSet(3).name = 'Step Irradiance'
      | sbobj.Groups(1).Name = 'Constant Irradiance'
      | sbobj.Groups(1).Signals(1).Name = 'Ir'
      | sbobj.Groups(1).Signals(1).XData = [0 1]
      | sbobj.Groups(1).Signals(1).YData = [1000 1000]
      | sbobj.Groups(1).Signals(2).Name = 'Temp'
      | sbobj.Groups(1).Signals(2).XData = [0 0.2 0.2 0.4 0.4 1]
      | sbobj.Groups(1).Signals(2).YData = [25 25 45 45 60 60]
      | sbobj.Groups(1).TimeRange = [0 1]
      | sbobj.Groups(2).Name = 'Ramp-up/down Irradiance'
      | sbobj.Groups(2).Signals(1).Name = 'Ir'
      | sbobj.Groups(2).Signals(1).XData = [0 0.3 0.3 0.4 0.4 0.5 0.5 1 2]
      | sbobj.Groups(2).Signals(1).YData = [1000 1000 800 795 600 600 400 395 395]
      | sbobj.Groups(2).Signals(2).Name = 'Temp'
      | sbobj.Groups(2).Signals(2).XData = [0 0.8 0.8 2]
      | sbobj.Groups(2).Signals(2).YData = [15 15 35 35]
      | sbobj.Groups(2).TimeRange = [0 2]
      | sbobj.Groups(3).Name = 'Step Irradiance'
      | sbobj.Groups(3).Signals(1).Name = 'Ir'
      | sbobj.Groups(3).Signals(1).XData = [0 0.252 0.252 2]
      | sbobj.Groups(3).Signals(1).YData = [600 600 1000 1000]
      | sbobj.Groups(3).Signals(2).Name = 'Temp'
      | sbobj.Groups(3).Signals(2).XData = [0 0.6 0.6 2]
      | sbobj.Groups(3).Signals(2).YData = [15 15 36.5 19.5]
      | sbobj.Groups(3).TimeRange = [0 2]
  Ir : Outport  Tag=STV Outport
  Temp : Outport  Tag=STV Outport  Port=2
  wires:
  FromWs/1 -> Demux/1
  Demux/1 -> Ir/1
  Demux/2 -> Temp/1

== system ALL_IN_ONE/Solar Panel3/Irradiance  ==
  Demux : Demux  Tag=STV Demux  Outputs=2
      settings: DisplayOption=none
  FromWs : FromWorkspace  Tag=STV FromWs  VariableName=tuvar
      SigBuilderData=|
      | common.afterFinalStr = 'Extrapolate'
      | common.sampleTime = '0'
      | dataSet(1).timeRange = [0 2]
      | dataSet(1).name = 'Constant Irradiance'
      | dataSet(2).timeRange = [0 2]
      | dataSet(2).name = 'Step Irradiance'
      | dataSet(3).timeRange = [0 1]
      | dataSet(3).name = 'Ramp-up/down Irradiance'
      | sbobj.Groups(1).Name = 'Constant Irradiance'
      | sbobj.Groups(1).Signals(1).Name = 'Ir'
      | sbobj.Groups(1).Signals(1).XData = [0 2]
      | sbobj.Groups(1).Signals(1).YData = [1000 1000]
      | sbobj.Groups(1).Signals(2).Name = 'Temp'
      | sbobj.Groups(1).Signals(2).XData = [0 1 1 2]
      | sbobj.Groups(1).Signals(2).YData = [0 0 1 1]
      | sbobj.Groups(1).TimeRange = [0 2]
      | sbobj.Groups(2).Name = 'Step Irradiance'
      | sbobj.Groups(2).Signals(1).Name = 'Ir'
      | sbobj.Groups(2).Signals(1).XData = [0 0.252 0.252 2]
      | sbobj.Groups(2).Signals(1).YData = [600 600 1000 1000]
      | sbobj.Groups(2).Signals(2).Name = 'Temp'
      | sbobj.Groups(2).Signals(2).XData = [0 1 1 2]
      | sbobj.Groups(2).Signals(2).YData = [0 0 1 1]
      | sbobj.Groups(2).TimeRange = [0 2]
      | sbobj.Groups(3).Name = 'Ramp-up/down Irradiance'
      | sbobj.Groups(3).Signals(1).Name = 'Ir'
      | sbobj.Groups(3).Signals(1).XData = [0 0.2 0.2 0.4 0.4 0.6 0.6 0.8 0.8 1]
      | sbobj.Groups(3).Signals(1).YData = [1000 1000 100 100 400 400 700 700 1000 1000]
      | sbobj.Groups(3).Signals(2).Name = 'Temp'
      | sbobj.Groups(3).Signals(2).XData = [0 1]
      | sbobj.Groups(3).Signals(2).YData = [25 25]
      | sbobj.Groups(3).TimeRange = [0 1]
  Ir : Outport  Tag=STV Outport
  Temp : Outport  Tag=STV Outport  Port=2
  wires:
  Demux/1 -> Ir/1
  FromWs/1 -> Demux/1
  Demux/2 -> Temp/1

== system ALL_IN_ONE/Solar Panel3/Temperature1 ==
  Demux : Demux  Tag=STV Demux  Outputs=2
      settings: DisplayOption=none
  FromWs : FromWorkspace  Tag=STV FromWs  VariableName=tuvar
      SigBuilderData=|
      | common.afterFinalStr = 'Extrapolate'
      | common.sampleTime = '0'
      | dataSet(1).timeRange = [0 1]
      | dataSet(1).name = 'Constant Irradiance'
      | dataSet(2).timeRange = [0 2]
      | dataSet(2).name = 'Ramp-up/down Irradiance'
      | dataSet(3).timeRange = [0 2]
      | dataSet(3).name = 'Step Irradiance'
      | sbobj.Groups(1).Name = 'Constant Irradiance'
      | sbobj.Groups(1).Signals(1).Name = 'Ir'
      | sbobj.Groups(1).Signals(1).XData = [0 1]
      | sbobj.Groups(1).Signals(1).YData = [996.86 996.86]
      | sbobj.Groups(1).Signals(2).Name = 'Temp'
      | sbobj.Groups(1).Signals(2).XData = [0 0.2 0.2 0.4 0.4 1]
      | sbobj.Groups(1).Signals(2).YData = [25 25 45 45 60 60]
      | sbobj.Groups(1).TimeRange = [0 1]
      | sbobj.Groups(2).Name = 'Ramp-up/down Irradiance'
      | sbobj.Groups(2).Signals(1).Name = 'Ir'
      | sbobj.Groups(2).Signals(1).XData = [0 0.3 0.3 0.4 0.4 0.5 0.5 1 2]
      | sbobj.Groups(2).Signals(1).YData = [1000 1000 800 795 600 600 400 395 395]
      | sbobj.Groups(2).Signals(2).Name = 'Temp'
      | sbobj.Groups(2).Signals(2).XData = [0 0.8 0.8 2]
      | sbobj.Groups(2).Signals(2).YData = [15 15 35 35]
      | sbobj.Groups(2).TimeRange = [0 2]
      | sbobj.Groups(3).Name = 'Step Irradiance'
      | sbobj.Groups(3).Signals(1).Name = 'Ir'
      | sbobj.Groups(3).Signals(1).XData = [0 0.252 0.252 2]
      | sbobj.Groups(3).Signals(1).YData = [600 600 1000 1000]
      | sbobj.Groups(3).Signals(2).Name = 'Temp'
      | sbobj.Groups(3).Signals(2).XData = [0 0.6 0.6 2]
      | sbobj.Groups(3).Signals(2).YData = [15 15 36.5 19.5]
      | sbobj.Groups(3).TimeRange = [0 2]
  Ir : Outport  Tag=STV Outport
  Temp : Outport  Tag=STV Outport  Port=2
  wires:
  FromWs/1 -> Demux/1
  Demux/1 -> Ir/1
  Demux/2 -> Temp/1

== matlab function ALL_IN_ONE/ML Algorithem/MATLAB Function1 ==
  data: Irr input; scaled_data output; Temp input; V_pv input; I_pv input
function scaled_data = scale_inputs(Irr, Temp, V_pv, I_pv)
    
    % EXACT MIN AND MAX VALUES FROM YOUR CSV
    min_vals = [100.0, 15.0, 3.70, 0.29];  
    max_vals = [1000.0, 60.0, 19.48, 2.80]; 
    
    raw_data = [Irr, Temp, V_pv, I_pv];
    scaled_data = zeros(1,4);
    
    for i = 1:4
        scaled_data(i) = (raw_data(i) - min_vals(i)) / (max_vals(i) - min_vals(i));
        if scaled_data(i) > 1.0; scaled_data(i) = 1.0;
        elseif scaled_data(i) < 0.0; scaled_data(i) = 0.0; end
    end
end

== matlab function ALL_IN_ONE/P & O algorithem/MATLAB Function ==
  data: V input; duty output; I input
function duty = PandO_Algorithm(V, I)
    % Stabilized P&O MPPT Algorithm
    % Includes Execution Delay and Deadband
    
    persistent V_old P_old D_old Loop_Counter;

    % Initialization
    if isempty(D_old)
        V_old = 0;
        P_old = 0;
        D_old = 0.29;   % Start near the expected 29% to reduce startup swing
        Loop_Counter = 0;
    end

    % --- TUNING PARAMETERS ---
    % 1. Step Size: Smaller steps reduce oscillation magnitude
    deltaD = 0.002;   
    
    % 2. Update Delay: How many simulation steps to wait before changing Duty.
    % Increase this if oscillation continues. (Try 500, 1000, or 2000)
    Update_Delay = 500; 
    
    % 3. Power Deadband: Ignore tiny power changes (noise)
    Power_Deadband = 0.2; % Watts

    % --- Code Execution ---
    P = V * I;
    Loop_Counter = Loop_Counter + 1;

    % CHECK: Only run P&O logic if the delay time has passed
    if Loop_Counter >= Update_Delay
        
        % Reset Counter
        Loop_Counter = 0;
        
        dP = P - P_old;
        dV = V - V_old;

        % Only change Duty if power change is real (larger than deadband)
        if abs(dP) > Power_Deadband
            if dP > 0
                % Power INCREASED
                if dV > 0
                    D_old = D_old - deltaD; % Left of MPP -> Decrease D (Increase V)
                else
                    D_old = D_old + deltaD; % Right of MPP -> Increase D (Decrease V)
                end
            else
                % Power DECREASED
                if dV > 0
                    D_old = D_old + deltaD; % Go back
                else
                    D_old = D_old - deltaD; % Go back
                end
            end
        end
        
        % Saturation Limits
        if D_old > 0.85
            D_old = 0.85;
        elseif D_old < 0.05
            D_old = 0.05;
        end
        
        % Update History only when we actually calculate
        V_old = V;
        P_old = P;
    end

    % Output the held Duty Cycle
    duty = D_old;
end

== matlab function ALL_IN_ONE/IC Algorithem/MATLAB Function ==
  data: V input; duty output; I input
function duty = IC_Algorithm(V, I)
% Incremental Conductance (INC) MPPT algorithm for a Boost Converter

% Declare persistent variables to hold previous step values across simulation steps
persistent V_prev I_prev D_prev;

% Initialize persistent variables on the first iteration
if isempty(V_prev)
    V_prev = 0;
    I_prev = 0;
    D_prev = 1; % Start with a 50% duty cycle
end

% --- Parameters to Tune ---
% Since your switching frequency is 10kHz, if this block runs at 10kHz, 
% deltaD should be very small to avoid oscillations. If you run this block 
% at a slower sampling rate (e.g., 100Hz), you can use a larger deltaD.
deltaD = 0.002;  % Step size for duty cycle (Tune this for your system)
D_max = 0.85;    % Maximum duty cycle limit to protect the converter
D_min = 0.15;    % Minimum duty cycle limit

% Prevent division by zero if V drops completely during startup
if V < 0.1
    V = 0.1;
end

% Calculate increments
dV = V - V_prev;
dI = I - I_prev;

% --- Incremental Conductance Core Logic ---
if dV == 0
    if dI == 0
        duty = D_prev; % No change, maintain current state
    elseif dI > 0
        % Irradiance increased. To find new MPP, increase V -> Decrease Duty
        duty = D_prev - deltaD; 
    else
        % Irradiance decreased. To find new MPP, decrease V -> Increase Duty
        duty = D_prev + deltaD; 
    end
else
    % Calculate instantaneous (G) and incremental (dG) conductance
    G = I / V;
    dG = dI / dV;
    
    % Use a small tolerance instead of exact equality for floating-point math
    tol = 0.4; 
    
    if abs(dG + G) < tol
        duty = D_prev; % Reached MPP
    elseif dG > -G
        % Operating point is Left of MPP -> Need to increase V -> Decrease Duty
        duty = D_prev - deltaD; 
    else
        % Operating point is Right of MPP -> Need to decrease V -> Increase Duty
        duty = D_prev + deltaD; 
    end
end

% --- Apply Duty Cycle Limits ---
if duty > D_max
    duty = D_max;
elseif duty < D_min
    duty = D_min;
end

% Update persistent variables for the next cycle
V_prev = V;
I_prev = I;
D_prev = duty;

end
